simulink model "AdaptiveThresholdSigmaDelta"  (R2020a)
settings: Solver=VariableStepAuto  StartTime=0.0  StopTime=10  RelTol=1e-3
undefined symbols (not defined in the file): DiscIntNeverNeededParam
libraries: dspswit3 x1, dspfdesign x1, simulink x1, hdlsllib x1
settings Model: Creator=diflo  LastModifiedBy=diflo

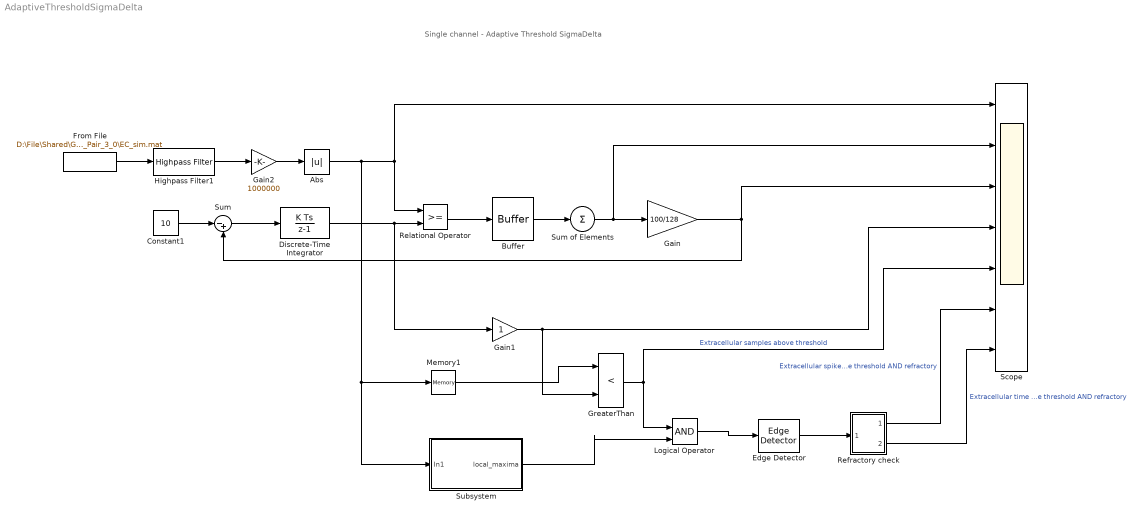
== system AdaptiveThresholdSigmaDelta ==
  note: Single channel - Adaptive Threshold SigmaDelta
  Abs : Abs
  Buffer : Buffer  N=128  OutputFrames=off
  Constant1 : Constant  Value=10  SampleTime=1/30000
  Discrete-Time Integrator : DiscreteIntegrator  gainval=0.1  SampleTime=1/30000  ICPrevOutput=DiscIntNeverNeededParam  ICPrevScaledInput=DiscIntNeverNeededParam
  Edge Detector : dspswit3/Edge Detector  InputProcessing=Columns as channels (frame based)
      settings: SourceProductBaseCode=DS
  From File : FromFile  FileName=D:\File\Shared\Google Drive\IIT - Neuroengineering\Project\WP1\Data\KampffLab\2014_11_25_Pair_3_0\EC_sim.mat  SampleTime=1/30000
  Gain : Gain  Gain=100/128
  Gain1 : Gain
  Gain2 : Gain  Gain=1000000
  GreaterThan : RelationalOperator  Operator=<  OutDataTypeStr=boolean  RndMeth=Simplest
  Highpass Filter1 : dspfdesign/Highpass Filter  FilterType=IIR  DesignForMinimumOrder=off  FilterOrder=3  StopbandFrequency=1  PassbandFrequency=300  StopbandAttenuation=80  PassbandRipple=0.1  InheritSampleRate=off  SampleRate=30000  SimulateUsing=Interpreted execution  roundingMode=Floor  coeffsDataTypeStr=fixdt(1,16)
  Logical Operator : Logic  IconShape=distinctive  AllPortsSameDT=off  OutDataTypeStr=boolean
  Memory1 : Memory  InheritSampleTime=on
  Refractory check : Subsystem
  Relational Operator : RelationalOperator  OutDataTypeStr=boolean
  Scope : Scope  NumInputPorts=7
  Subsystem : Subsystem
  Sum : Sum  Inputs=|-+
  Sum of Elements : Sum  Inputs=+
  wires:
  Abs/1 -> Subsystem/1(In1), Memory1/1, Scope/1, Relational Operator/1
  Discrete-Time Integrator/1 -> Gain1/1, Relational Operator/2
  Sum/1 -> Discrete-Time Integrator/1
  Constant1/1 -> Sum/1
  Relational Operator/1 -> Buffer/1
  Buffer/1 -> Sum of Elements/1
  Sum of Elements/1 -> Scope/2, Gain/1
  Gain/1 -> Sum/2, Scope/3
  Gain1/1 -> Scope/4, GreaterThan/2
  From File/1 -> Highpass Filter1/1
  Highpass Filter1/1 -> Gain2/1
  Gain2/1 -> Abs/1
  Memory1/1 -> GreaterThan/1
  Subsystem/1(local_maxima) -> Logical Operator/2
  GreaterThan/1 -> Scope/5, Logical Operator/1  "Extracellular samples above threshold"
  Edge Detector/1 -> Refractory check/1("   ")
  Logical Operator/1 -> Edge Detector/1
  Refractory check/1(" ") -> Scope/6  "Extracellular spikes above threshold AND refractory"
  Refractory check/2(Output) -> Scope/7  "Extracellular time since last spike above threshold AND refractory"

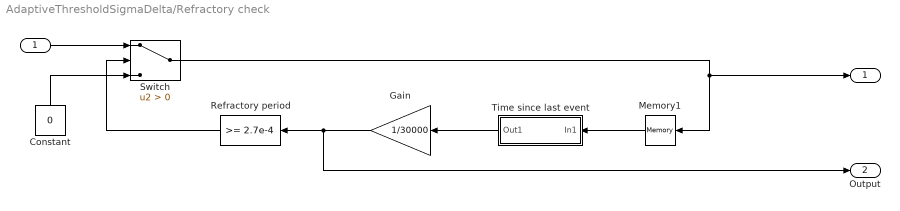
== system AdaptiveThresholdSigmaDelta/Refractory check ==
  "   " : Inport
  Constant : Constant  Value=0
  Gain : Gain  Gain=1/30000  ParamDataTypeStr=double
  Memory1 : Memory  InheritSampleTime=on
  Refractory period : simulink/Logic and Bit Operations/Compare To Constant  relop=>=  const=2.7e-4  OutDataTypeStr=boolean
  Switch : Switch  Criteria=u2 > Threshold
  Time since last event : Subsystem
  " " : Outport
  Output : Outport  Port=2
  wires:
  "   "/1 -> Switch/1
  Memory1/1 -> Time since last event/1(In1)
  Time since last event/1(Out1) -> Gain/1
  Constant/1 -> Switch/3
  Gain/1 -> Refractory period/1, Output/1
  Switch/1 -> " "/1, Memory1/1
  Refractory period/1 -> Switch/2

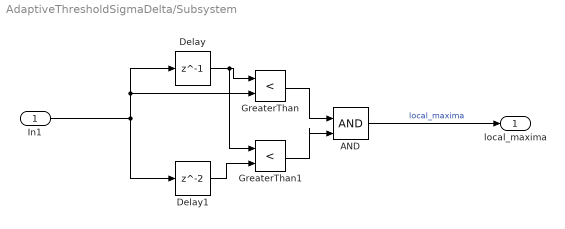
== system AdaptiveThresholdSigmaDelta/Subsystem ==
  In1 : Inport
  AND : Logic  IconShape=distinctive  AllPortsSameDT=off  OutDataTypeStr=boolean
  Delay : Delay  DelayLength=1  SampleTime=1/30000
  Delay1 : Delay  SampleTime=1/30000
  GreaterThan : RelationalOperator  Operator=<  OutDataTypeStr=boolean  RndMeth=Simplest
  GreaterThan1 : RelationalOperator  Operator=<  OutDataTypeStr=boolean  RndMeth=Simplest
  local_maxima : Outport
  wires:
  Delay/1 -> GreaterThan1/1, GreaterThan/1
  In1/1 -> Delay/1, GreaterThan/2, Delay1/1
  GreaterThan/1 -> AND/1
  GreaterThan1/1 -> AND/2
  AND/1 -> local_maxima/1  "local_maxima"
  Delay1/1 -> GreaterThan1/2

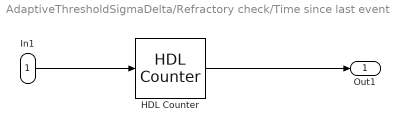
== system AdaptiveThresholdSigmaDelta/Refractory check/Time since last event ==
  In1 : Inport
  HDL Counter : hdlsllib/Sources/HDL Counter  CountType=Free running  CountInit=1  CountStep=1  CountMax=25  CountFromType=Initial value  CountFrom=1  CountResetPort=on  CountLoadPort=off  CountEnbPort=off  CountDirPort=off  CountDataType=Unsigned  CountWordLen=32  CountFracLen=0  CountSampTime=1
  Out1 : Outport
  wires:
  In1/1 -> HDL Counter/1
  HDL Counter/1 -> Out1/1
